simulink model "Contol_loop_v1"  (R2023b)
settings: Solver=VariableStepAuto  StartTime=0.0  StopTime=10.0  RelTol=1e-3
model mask{J2=I1, J1=I2, m2=M1, m1=M2, r1=r1, r2=r2, g=g}
  mask prompts: J2 "I1:"; J1 "I2:"; m2 "M1:"; m1 "M2:"
model workspace (MAT data in the model file):
  J1 = 0
  J2 = 0
  g = 0
  m1 = 0
  m2 = 0
  r1 = 0
  r2 = 0
values from neighbouring files (symbols this model uses):
  C = [-p2*sin(q2)*dq1, -2*p2*sin(q2)*dq1 ... (first row only)    [Control_v1.m]
undefined symbols (not defined in the file or in its folder): a1, b1, c1, D, d1, K, n
settings Model: ParameterArgumentNames=J1,J2,g,m1,m2,r1,r2  Creator=anthe  LastModifiedBy=anthe

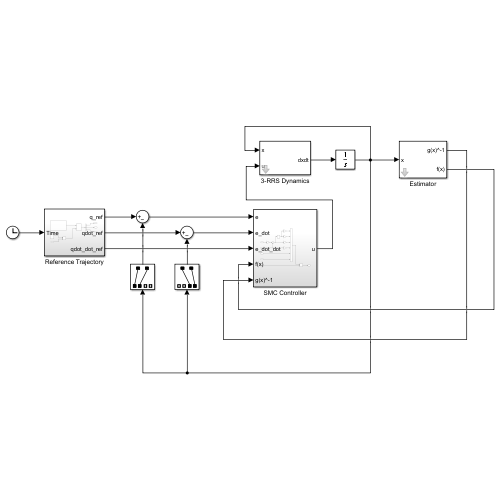
[thumbnail: Simulink's stored preview of the top-level diagram]
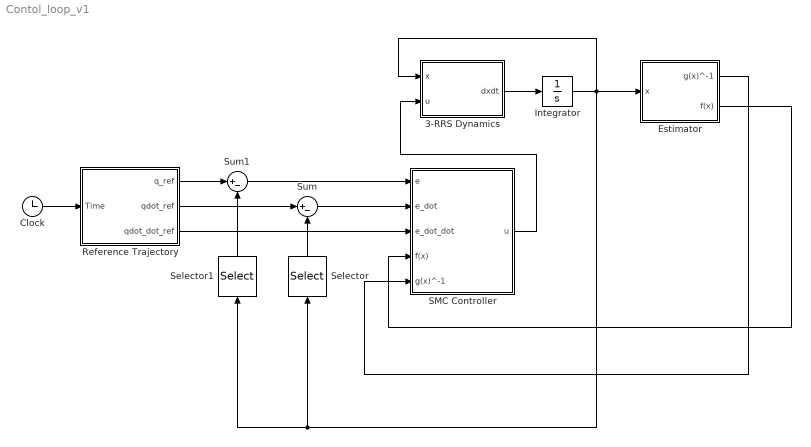
== system Contol_loop_v1 ==
  3-RRS Dynamics : Subsystem  mask{MassLink1=0, MassLink2=0, InertialMatrix1=0, InertialMatrix2=0, LengthLink1=0, LengthLink2=0, Gravity=0}
      mask prompts: MassLink1 "m1"; MassLink2 "m2"; InertialMatrix1 "J1"; InertialMatrix2 "J2"; LengthLink1 "r1"; LengthLink2 "r2"; Gravity "g"
  Clock : Clock
  Estimator : Subsystem  mask{MassLink1=0, MassLink2=0, LengthLink1=0, LengthLink2=0, InertialMatrix1=0, InertialMatrix2=0, Gravity=0}
      mask prompts: MassLink1 "m1_E"; MassLink2 "m2_E"; LengthLink1 "r1_E"; LengthLink2 "r2_E"; InertialMatrix1 "J1_E"; InertialMatrix2 "J2_E"; Gravity "g"
  Integrator : Integrator
  Reference Trajectory : Subsystem
  SMC Controller : Subsystem
  Selector : Selector  InputPortWidth=4  IndexOptions=Index vector (dialog)  Indices=[3 4]  OutputSizes=1
  Selector1 : Selector  InputPortWidth=4  IndexOptions=Index vector (dialog)  Indices=[1 2]  OutputSizes=1
  Sum : Sum  Inputs=|+-
  Sum1 : Sum  Inputs=|+-
  wires:
  3-RRS Dynamics/1(dxdt) -> Integrator/1
  SMC Controller/1(u) -> 3-RRS Dynamics/2(u)
  Estimator/2(f(x)) -> SMC Controller/4(f(x))
  Estimator/1(g(x)^-1) -> SMC Controller/5(g(x)^-1)
  Clock/1 -> Reference Trajectory/1(Time)
  Selector/1 -> Sum/2
  Selector1/1 -> Sum1/2
  Reference Trajectory/1(q_ref) -> Sum1/1
  Sum1/1 -> SMC Controller/1(e)
  Reference Trajectory/2(qdot_ref) -> Sum/1
  Sum/1 -> SMC Controller/2(e_dot)
  Reference Trajectory/3(qdot_dot_ref) -> SMC Controller/3(e_dot_dot)
  Integrator/1 -> Estimator/1(x), Selector/1, Selector1/1, 3-RRS Dynamics/1(x)

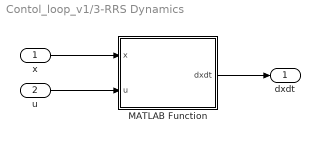
== system Contol_loop_v1/3-RRS Dynamics ==
  x : Inport
  u : Inport  Port=2
  MATLAB Function : MATLAB Function  TreatAsAtomicUnit=on
  dxdt : Outport
  wires:
  x/1 -> MATLAB Function/1(x)
  u/1 -> MATLAB Function/2(u)
  MATLAB Function/1(dxdt) -> dxdt/1

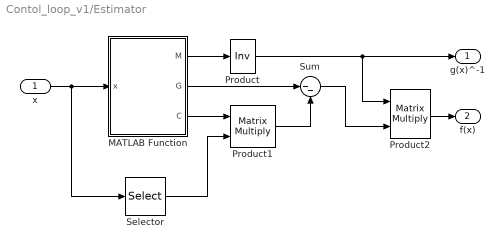
== system Contol_loop_v1/Estimator ==
  x : Inport
  MATLAB Function : MATLAB Function  TreatAsAtomicUnit=on
  Product : Product  Inputs=/  Multiplication=Matrix(*)
  Product1 : Product  Multiplication=Matrix(*)
  Product2 : Product  Inputs=**  Multiplication=Matrix(*)
  Selector : Selector  InputPortWidth=4  IndexOptions=Index vector (dialog)  Indices=[3 4]  OutputSizes=1
  Sum : Sum  Inputs=|--
  g(x)^-1 : Outport
  f(x) : Outport  Port=2
  wires:
  x/1 -> Selector/1, MATLAB Function/1(x)
  Product/1 -> Product2/1, g(x)^-1/1
  MATLAB Function/1(M) -> Product/1
  MATLAB Function/3(C) -> Product1/1
  MATLAB Function/2(G) -> Sum/1
  Product1/1 -> Sum/2
  Selector/1 -> Product1/2
  Product2/1 -> f(x)/1
  Sum/1 -> Product2/2

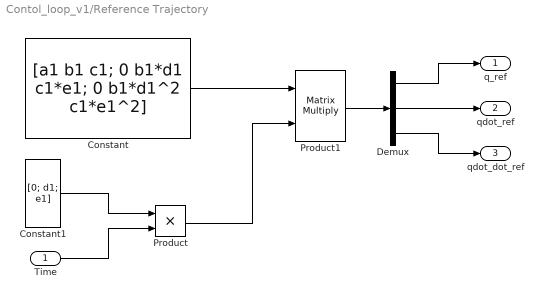
== system Contol_loop_v1/Reference Trajectory ==
  Time : Inport
  Constant : Constant  Value=[a1 b1 c1; 0 b1*d1 c1*e1; 0 b1*d1^2 c1*e1^2]  VectorParams1D=off
  Constant1 : Constant  Value=[0; d1; e1]  VectorParams1D=off
  Demux : Demux  Outputs=3
  Product : Product
  Product1 : Product  Multiplication=Matrix(*)
  q_ref : Outport
  qdot_ref : Outport  Port=2
  qdot_dot_ref : Outport  Port=3
  wires:
  Constant1/1 -> Product/1
  Time/1 -> Product/2
  Constant/1 -> Product1/1
  Product/1 -> Product1/2
  Product1/1 -> Demux/1
  Demux/1 -> q_ref/1
  Demux/2 -> qdot_ref/1
  Demux/3 -> qdot_dot_ref/1

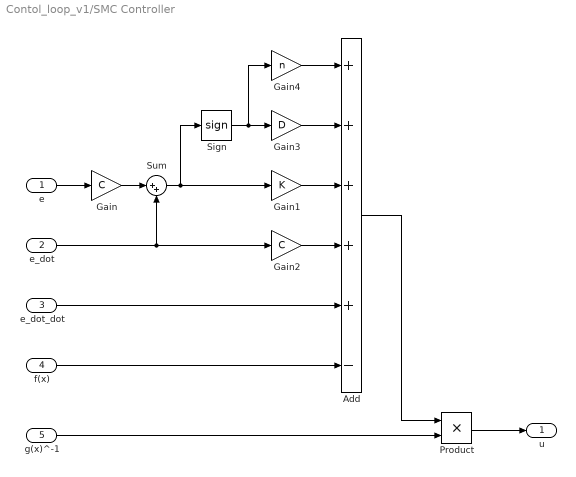
== system Contol_loop_v1/SMC Controller ==
  e : Inport
  e_dot : Inport  Port=2
  e_dot_dot : Inport  Port=3
  f(x) : Inport  Port=4
  g(x)^-1 : Inport  Port=5
  Add : Sum  Inputs=+++++-
  Gain : Gain  Gain=C
  Gain1 : Gain  Gain=K
  Gain2 : Gain  Gain=C
  Gain3 : Gain  Gain=D
  Gain4 : Gain  Gain=n
  Product : Product
  Sign : Signum
  Sum : Sum  Inputs=|++
  u : Outport
  wires:
  e/1 -> Gain/1
  Gain/1 -> Sum/1
  e_dot/1 -> Sum/2, Gain2/1
  Sum/1 -> Sign/1, Gain1/1
  Gain1/1 -> Add/3
  Gain2/1 -> Add/4
  Sign/1 -> Gain4/1, Gain3/1
  Gain3/1 -> Add/2
  Gain4/1 -> Add/1
  e_dot_dot/1 -> Add/5
  f(x)/1 -> Add/6
  Product/1 -> u/1
  g(x)^-1/1 -> Product/2
  Add/1 -> Product/1

== matlab function Contol_loop_v1/Estimator/MATLAB Function ==
  data: x input; M output; G output; C output
function [M, G, C] = fcn(x)

param.m1 = m1_E; % Mass 1
param.m2 = m2_E; % Mass 2
param.r1 = r1_E; % Link length 1
param.r2 = r2_E; % Link length 2
param.J1 = J1_E; % Inertia 1
param.J2 = J2_E; % Inertia 2
param.g  = g;  % Gravity constant2

M = zeros(2,2,'like', x);
C = zeros(2,2,'like', x);
G = zeros(2,1,'like', x);

[~, M, C, G] = Control_v1(x, zeros(2,1), param);

== matlab function Contol_loop_v1/3-RRS Dynamics/MATLAB Function ==
  data: x input; u input; dxdt output
function dxdt = fcn(x, u)
param.m1 = m1; % Mass 1
param.m2 = m2; % Mass 2
param.r1 = r1; % Link length 1
param.r2 = r2; % Link length 2
param.J1 = J1; % Inertia 1
param.J2 = J2; % Inertia 2
param.g  = g;  % Gravity constant

dxdt = zeros(4,1,'like', x);
dxdt = Control_v1(x, u, param);

end
